simulink model "modules_intentions"  (R2017a)
settings: Solver=ode4  StartTime=0.0  StopTime=time_stop  FixedStep=time_step  RelTol=1e-3
undefined symbols (not defined in the file or in its folder): beta, Delta_guidance, Delta_matrix, eta_initial, initial_desired_psi_vector, initial_desired_u_vector, initial_next_waypoint_indexes, initial_obstacle_ship_states, initial_obstacle_ship_states_dot, initial_reference_psi_vector, initial_reference_u_vector, initial_SBMPC_desired_psi_vector, initial_SBMPC_desired_u_vector, initial_SBMPC_next_waypoint_indexes, initial_SBMPC_obstacle_ship_states, initial_SBMPC_obstacle_ship_states_dot, initial_SBMPC_reference_psi_vector, initial_SBMPC_reference_u_vector, initial_SBMPC_x_d_psi_matrix, initial_SBMPC_x_d_u_matrix, initial_state, initial_x_d_psi_matrix, initial_x_d_u_matrix, K_sway, K_yaw, Kp_feedback_linearization, kp_heading, Nmax, nu_initial, num_obs_ship_waypoints, num_prediction_time_steps, number_of_control_behaviors, number_of_obstacle_ships, number_of_SBMPC_obstacle_ships, obs_speed_between_waypoints, obstacle_waypoint_matrix, Omega_matrix, own_ship_reference_psi_init, own_ship_reference_speed, psi, Psi_init, radius_of_acceptance, SBMPC_obs_speed_between_waypoints, SBMPC_obstacle_waypoint_matrix, seconds_between_prediction, state_vector_init, T, T_k_surge, T_k_sway, T_k_yaw, T_s, T_waypoints, time_step, tsamp, U, U_init, V_init, waypoints_obstacle_ships, waypoints_own_ship, Xmax ... (+1)
(part 2 of 6)

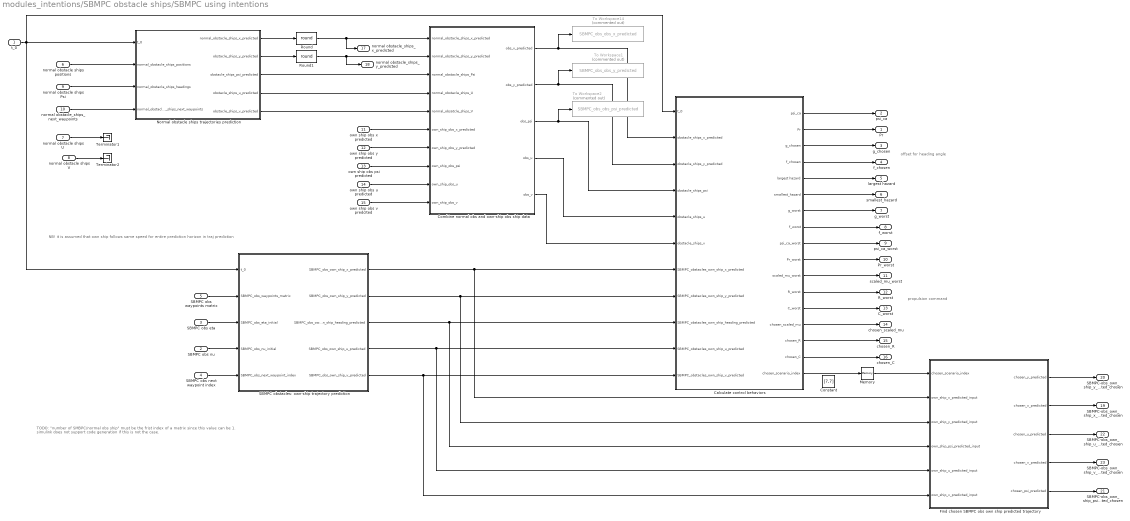
== system modules_intentions/SBMPC obstacle ships/SBMPC using intentions  ==
  note: TODO: "number of SMBPC/normal obs ship" must be the frist index of a matrix since this value can be 1. simulink
      | does not support code generation if this is not the case.
  note: propulsion command
  note: offset for heading angle
  note: NB! it is assumed that own ship follows same speed for entire prediction horizon in traj prediction
  t_0 : Inport
  SBMPC obs nu : Inport  Port=2
  SBMPC obs eta : Inport  Port=3
  SBMPC obs next waypoint index : Inport  Port=4
  "SBMPC obs waypoints matrix " : Inport  Port=5
  normal obstacle ships positions : Inport  Port=6
  normal obstacle ships U : Inport  Port=7
  normal obstacle ships V : Inport  Port=8
  normal obstacle ships Psi : Inport  Port=9
  normal obstacle_ships_next_waypoints : Inport  Port=10
  own ship obs x predicted : Inport  Port=11  SampleTime=time_step
  own ship obs y predicted : Inport  Port=12  SampleTime=time_step
  own ship obs psi predicted : Inport  Port=13
  own ship obs u predicted : Inport  Port=14
  own ship obs v predcited : Inport  Port=15
  Calculate control behaviors : Subsystem
  "Combine normal obs and own-ship obs ship data " : MATLAB Function  TreatAsAtomicUnit=on
  Constant : Constant  Value=[7,7]  VectorParams1D=off
  Find chosen SBMPC obs own ship predicted trajectory : MATLAB Function  TreatAsAtomicUnit=on
  Memory : Memory  X0=7
  Normal obstacle ships trajectories prediction : Subsystem
  Round : Rounding  Operator=round
  Round1 : Rounding  Operator=round
  SBMPC obstacles: own-ship trajectory prediction : Subsystem
  Terminator1 : Terminator
  Terminator2 : Terminator
  To Workspace1 : ToWorkspace  Commented=on  VariableName=SBMPC_obs_obs_y_predicted  SaveFormat=Structure With Time  SampleTime=tsamp
      settings: Save2DSignal=2-D array (concatenate along first dimension)
  To Workspace14 : ToWorkspace  Commented=on  VariableName=SBMPC_obs_obs_x_predicted  SaveFormat=Structure With Time  SampleTime=tsamp
      settings: Save2DSignal=2-D array (concatenate along first dimension)
  To Workspace2 : ToWorkspace  Commented=on  VariableName=SBMPC_obs_obs_psi_predicted  SaveFormat=Structure With Time  SampleTime=tsamp
      settings: Save2DSignal=2-D array (concatenate along first dimension)
  Pr : Outport
  psi_ca : Outport  Port=2
  "g_chosen " : Outport  Port=3  SampleTime=time_step
  f_chosen : Outport  Port=4  SampleTime=time_step
  largest hazard : Outport  Port=5  SampleTime=time_step
  smallest_hazard : Outport  Port=6  SampleTime=time_step
  "g_worst " : Outport  Port=7  SampleTime=time_step
  f_worst : Outport  Port=8  SampleTime=time_step
  psi_ca_worst : Outport  Port=9  SampleTime=time_step
  Pr_worst : Outport  Port=10  SampleTime=time_step
  scaled_mu_worst : Outport  Port=11  SampleTime=time_step
  R_worst : Outport  Port=12  SampleTime=time_step
  C_worst : Outport  Port=13  SampleTime=time_step
  chosen_scaled_mu : Outport  Port=14  SampleTime=time_step
  chosen_R : Outport  Port=15  SampleTime=time_step
  chosen_C : Outport  Port=16  SampleTime=time_step
  normal obstacle_ships_x_predicted : Outport  Port=17  SampleTime=time_step
  "normal obstacle_ships_y_predicted " : Outport  Port=18  SampleTime=time_step
  SBMPC-obs_own_ship_x_predicted_chosen : Outport  Port=19  SampleTime=time_step
  SBMPC-obs_own_ship_y_predicted_chosen : Outport  Port=20  SampleTime=time_step
  SBMPC-obs_own_ship_psi_predicted_chosen : Outport  Port=21  SampleTime=time_step
  SBMPC-obs_own_ship_u_predicted_chosen : Outport  Port=22  SampleTime=time_step
  SBMPC-obs_own_ship_v_predicted_chosen : Outport  Port=23  SampleTime=time_step
  wires:
  "SBMPC obs waypoints matrix "/1 -> SBMPC obstacles: own-ship trajectory prediction/2(SBMPC_obs_waypoints_matrix)
  SBMPC obs eta/1 -> SBMPC obstacles: own-ship trajectory prediction/3("SBMPC_obs_eta_initial ")
  SBMPC obs nu/1 -> SBMPC obstacles: own-ship trajectory prediction/4(SBMPC_obs_nu_initial)
  SBMPC obs next waypoint index/1 -> SBMPC obstacles: own-ship trajectory prediction/5(SBMPC_obs_next_waypoint_index)
  t_0/1 -> Calculate control behaviors/1(t_0), Normal obstacle ships trajectories prediction/1(t_0), SBMPC obstacles: own-ship trajectory prediction/1(t_0)
  normal obstacle ships positions/1 -> Normal obstacle ships trajectories prediction/2(normal_obstacle_ships_positions)
  normal obstacle ships Psi/1 -> Normal obstacle ships trajectories prediction/3(normal_obstacle_ships_headings)
  SBMPC obstacles: own-ship trajectory prediction/5("SBMPC_obs_own_ship_v_predicted ") -> Find chosen SBMPC obs own ship predicted trajectory/6(own_ship_v_predicted_input), Calculate control behaviors/11("SBMPC_obstacles_own_ship_v_predicted ")
  SBMPC obstacles: own-ship trajectory prediction/3(SBMPC_obs_own_ship_heading_predicted) -> Calculate control behaviors/9("SBMPC_obstacles_own_ship_heading_predicted "), Find chosen SBMPC obs own ship predicted trajectory/4(own_ship_psi_predicted_input)
  Calculate control behaviors/2(Pr) -> Pr/1
  Calculate control behaviors/1(psi_ca) -> psi_ca/1
  normal obstacle_ships_next_waypoints/1 -> Normal obstacle ships trajectories prediction/4(normal_obstacle_ships_next_waypoints)
  Calculate control behaviors/16(chosen_C) -> chosen_C/1
  Calculate control behaviors/15(chosen_R) -> chosen_R/1
  Calculate control behaviors/14(chosen_scaled_mu) -> chosen_scaled_mu/1
  Calculate control behaviors/13(C_worst) -> C_worst/1
  Calculate control behaviors/12(R_worst) -> R_worst/1
  Calculate control behaviors/11(scaled_mu_worst) -> scaled_mu_worst/1
  Calculate control behaviors/10(Pr_worst) -> Pr_worst/1
  Calculate control behaviors/9(psi_ca_worst) -> psi_ca_worst/1
  Calculate control behaviors/8(f_worst) -> f_worst/1
  Calculate control behaviors/7("g_worst ") -> "g_worst "/1
  Calculate control behaviors/6(smallest_hazard) -> smallest_hazard/1
  Calculate control behaviors/5(largest hazard) -> largest hazard/1
  Calculate control behaviors/4(f_chosen) -> f_chosen/1
  Calculate control behaviors/3("g_chosen ") -> "g_chosen "/1
  "Combine normal obs and own-ship obs ship data "/5(obs_v) -> Calculate control behaviors/6(obstacle_ships_v)
  "Combine normal obs and own-ship obs ship data "/4(obs_u) -> Calculate control behaviors/5(obstacle_ships_u)
  "Combine normal obs and own-ship obs ship data "/3(obs_psi) -> To Workspace2/1, Calculate control behaviors/4(obstacle_ships_psi)
  "Combine normal obs and own-ship obs ship data "/2(obs_y_predicted) -> To Workspace1/1, Calculate control behaviors/3("obstacle_ships_y_predicted ")
  "Combine normal obs and own-ship obs ship data "/1(obs_x_predicted) -> To Workspace14/1, Calculate control behaviors/2(obstacle_ships_x_predicted)
  own ship obs x predicted/1 -> "Combine normal obs and own-ship obs ship data "/6(own_ship_obs_x_predicted)
  own ship obs y predicted/1 -> "Combine normal obs and own-ship obs ship data "/7(own_ship_obs_y_predicted)
  own ship obs psi predicted/1 -> "Combine normal obs and own-ship obs ship data "/8(own_ship_obs_psi)
  own ship obs u predicted/1 -> "Combine normal obs and own-ship obs ship data "/9(own_ship_obs_u)
  own ship obs v predcited/1 -> "Combine normal obs and own-ship obs ship data "/10(own_ship_obs_v)
  SBMPC obstacles: own-ship trajectory prediction/1(SBMPC_obs_own_ship_x_predicted) -> Find chosen SBMPC obs own ship predicted trajectory/2(own_ship_x_predicted_input), Calculate control behaviors/7(SBMPC_obstacles_own_ship_x_predicted)
  SBMPC obstacles: own-ship trajectory prediction/2(SBMPC_obs_own_ship_y_predicted) -> Find chosen SBMPC obs own ship predicted trajectory/3(own_ship_y_predicted_input), Calculate control behaviors/8(SBMPC_obstacles_own_ship_y_predicted)
  SBMPC obstacles: own-ship trajectory prediction/4(SBMPC_obs_own_ship_u_predicted) -> Find chosen SBMPC obs own ship predicted trajectory/5(own_ship_u_predicted_input), Calculate control behaviors/10(SBMPC_obstacles_own_ship_u_predicted)
  Memory/1 -> Find chosen SBMPC obs own ship predicted trajectory/1(chosen_scenario_index)
  Find chosen SBMPC obs own ship predicted trajectory/1(chosen_y_predicted) -> SBMPC-obs_own_ship_y_predicted_chosen/1
  Find chosen SBMPC obs own ship predicted trajectory/2(chosen_x_predicted) -> SBMPC-obs_own_ship_x_predicted_chosen/1
  Find chosen SBMPC obs own ship predicted trajectory/3(chosen_u_predicted) -> SBMPC-obs_own_ship_u_predicted_chosen/1
  Find chosen SBMPC obs own ship predicted trajectory/4(chosen_v_predicted) -> SBMPC-obs_own_ship_v_predicted_chosen/1
  Find chosen SBMPC obs own ship predicted trajectory/5(chosen_psi_predicted) -> SBMPC-obs_own_ship_psi_predicted_chosen/1
  Normal obstacle ships trajectories prediction/2(obstacle_ships_y_predicted) -> Round1/1
  Normal obstacle ships trajectories prediction/3(obstacle_ships_psi_predicted) -> "Combine normal obs and own-ship obs ship data "/3(normal_obstacle_ships_Psi)
  Normal obstacle ships trajectories prediction/4(obstacle_ships_u_predicted) -> "Combine normal obs and own-ship obs ship data "/4(normal_obstacle_ships_U)
  Normal obstacle ships trajectories prediction/5(obstacle_ships_v_predicted) -> "Combine normal obs and own-ship obs ship data "/5(normal_obsatcle_ships_V)
  Normal obstacle ships trajectories prediction/1(normal_obstacle_ships_x_predicted) -> Round/1
  normal obstacle ships U/1 -> Terminator1/1
  normal obstacle ships V/1 -> Terminator2/1
  Calculate control behaviors/17(chosen_scenario_index) -> Memory/1
  Round/1 -> normal obstacle_ships_x_predicted/1, "Combine normal obs and own-ship obs ship data "/1(normal_obstacle_ships_x_predicted)
  Round1/1 -> "normal obstacle_ships_y_predicted "/1, "Combine normal obs and own-ship obs ship data "/2(normal_obstacle_ships_y_predicted)

== system modules_intentions/SBMPC obstacle ships/guidance  ==
  state matrix : Inport
  "waypoints matrix " : Inport  Port=2
  SBMPC obstacle waypoint guidance : MATLAB Function  TreatAsAtomicUnit=on
  SBMPC reference u vector : MATLAB Function  TreatAsAtomicUnit=on
  Scope : Scope
  Scope1 : Scope
  Scope2 : Scope
  "reference psi " : Outport
  reference u vector : Outport  Port=2
  "next_waypoints_indexes " : Outport  Port=3
  wires:
  "waypoints matrix "/1 -> SBMPC obstacle waypoint guidance/1(SBMPC_obstacle_waypoints)
  state matrix/1 -> SBMPC obstacle waypoint guidance/2(state_matrix)
  SBMPC obstacle waypoint guidance/1(reference_psi_vector) -> "reference psi "/1, Scope/1
  SBMPC reference u vector/1(u_vector) -> Scope2/1, reference u vector/1
  SBMPC obstacle waypoint guidance/2(next_waypoints_indexes) -> SBMPC reference u vector/1(next_waypoints_indexes), Scope1/1, "next_waypoints_indexes "/1

== system modules_intentions/SBMPC obstacle ships/reference model for psi ==
  note: row vector
  note: row vector
  reference psi vector : Inport
  "SBMPC psi reference model " : MATLAB Function  TreatAsAtomicUnit=on
  Scope3 : Scope  NumInputPorts=2
  To Workspace : ToWorkspace  VariableName=SBMPC_obstacle_ships_reference_psi_vector  SampleTime=tsamp
      settings: Save2DSignal=2-D array (concatenate along first dimension)
  To Workspace1 : ToWorkspace  VariableName=SBMPC_obstacle_ships_desired_psi_vector  SampleTime=tsamp
      settings: Save2DSignal=2-D array (concatenate along first dimension)
  "desired psi vector " : Outport
  wires:
  "SBMPC psi reference model "/1(desired_psi_vector) -> Scope3/1, To Workspace1/1, "desired psi vector "/1
  reference psi vector/1 -> Scope3/2, To Workspace/1, "SBMPC psi reference model "/1(reference_psi_vector)

== system modules_intentions/SBMPC obstacle ships/reference model for u ==
  note: row vector
  note: row vector
  "reference u vector " : Inport
  SBMPC obstacle ships reference model u : MATLAB Function  TreatAsAtomicUnit=on
  To Workspace : ToWorkspace  VariableName=SBMPC_obstacle_ships_reference_u_vector  SampleTime=tsamp
      settings: Save2DSignal=2-D array (concatenate along first dimension)
  To Workspace1 : ToWorkspace  VariableName=SBMPC_obstacle_ships_desired_u_vector  SampleTime=tsamp
      settings: Save2DSignal=2-D array (concatenate along first dimension)
  desired_u_vector : Outport
  wires:
  "reference u vector "/1 -> To Workspace/1, SBMPC obstacle ships reference model u/1(reference_u_vetor)
  SBMPC obstacle ships reference model u/1(desired_u_vector) -> To Workspace1/1, desired_u_vector/1

== system modules_intentions/normal obstacle ships/guidance  ==
  state matrix : Inport
  "waypoints matrix " : Inport  Port=2
  MATLAB Function1 : MATLAB Function  TreatAsAtomicUnit=on
  Scope : Scope
  Scope1 : Scope
  Scope2 : Scope
  obstacle waypoint guidance : MATLAB Function  TreatAsAtomicUnit=on
  "reference psi " : Outport
  reference u vector : Outport  Port=2
  "next_waypoints_indexes " : Outport  Port=3
  wires:
  "waypoints matrix "/1 -> obstacle waypoint guidance/1(obstacle_waypoints)
  state matrix/1 -> obstacle waypoint guidance/2(state_matrix)
  obstacle waypoint guidance/1(reference_psi_vector) -> "reference psi "/1, Scope/1
  MATLAB Function1/1(u_vector) -> Scope2/1, reference u vector/1
  obstacle waypoint guidance/2(next_waypoints_indexes) -> MATLAB Function1/1(next_waypoints_indexes), Scope1/1, "next_waypoints_indexes "/1

== system modules_intentions/normal obstacle ships/reference model for psi ==
  note: row vector
  note: row vector
  reference psi vector : Inport
  Scope3 : Scope  NumInputPorts=2
  To Workspace : ToWorkspace  VariableName=obstacle_ships_reference_psi_vector  SampleTime=tsamp
      settings: Save2DSignal=2-D array (concatenate along first dimension)
  To Workspace1 : ToWorkspace  VariableName=obstacle_ships_desired_psi_vector  SampleTime=tsamp
      settings: Save2DSignal=2-D array (concatenate along first dimension)
  "psi reference model " : MATLAB Function  TreatAsAtomicUnit=on
  "desired psi vector " : Outport
  wires:
  "psi reference model "/1(desired_psi_vector) -> Scope3/1, To Workspace1/1, "desired psi vector "/1
  reference psi vector/1 -> Scope3/2, To Workspace/1, "psi reference model "/1(reference_psi_vector)

== system modules_intentions/normal obstacle ships/reference model for u ==
  note: row vector
  note: row vector
  "reference u vector " : Inport
  MATLAB Function1 : MATLAB Function  TreatAsAtomicUnit=on
  To Workspace : ToWorkspace  VariableName=obstacle_ships_reference_u_vector  SampleTime=tsamp
      settings: Save2DSignal=2-D array (concatenate along first dimension)
  To Workspace1 : ToWorkspace  VariableName=obstacle_ships_desired_u_vector  SampleTime=tsamp
      settings: Save2DSignal=2-D array (concatenate along first dimension)
  desired_u_vector : Outport
  wires:
  "reference u vector "/1 -> To Workspace/1, MATLAB Function1/1(reference_u_vetor)
  MATLAB Function1/1(desired_u_vector) -> To Workspace1/1, desired_u_vector/1

== system modules_intentions/Own-ship/Own-ship PSV/PSV ==
  desired_nu : Inport
  desired_psi : Inport  Port=2
  Pr : Inport  Port=3
  psi_ca : Inport  Port=4
  Demux : Demux  Outputs=6
  Mux : Mux  Inputs=3
  PSV model : MATLAB Function  TreatAsAtomicUnit=on
  Terminator : Terminator
  To Workspace : ToWorkspace  VariableName=tau  SampleTime=tsamp
      settings: Save2DSignal=2-D array (concatenate along first dimension)
  state : Outport
  x : Outport  Port=2
  y : Outport  Port=3
  psi : Outport  Port=4
  u : Outport  Port=5
  v : Outport  Port=6
  r : Outport  Port=7
  wires:
  Demux/4 -> u/1, Mux/1
  Mux/1 -> Terminator/1  "nu"
  PSV model/1(state) -> Demux/1, state/1
  Demux/5 -> v/1, Mux/2
  Demux/2 -> y/1
  Demux/6 -> r/1, Mux/3
  Demux/1 -> x/1
  Demux/3 -> psi/1
  desired_psi/1 -> PSV model/4(desired_psi)
  desired_nu/1 -> PSV model/3(desired_nu)
  PSV model/2(tau) -> To Workspace/1
  psi_ca/1 -> PSV model/2(psi_ca)
  Pr/1 -> PSV model/1(Pr)

== system modules_intentions/Own-ship/Own-ship PSV/derivative ==
  desired_nu : Inport
  Memory2 : Memory
  vector derivative : MATLAB Function  TreatAsAtomicUnit=on
  desired_nu_dot : Outport
  wires:
  Memory2/1 -> vector derivative/2(x_previous)
  desired_nu/1 -> Memory2/1, vector derivative/1(x)
  vector derivative/1(derivative) -> desired_nu_dot/1

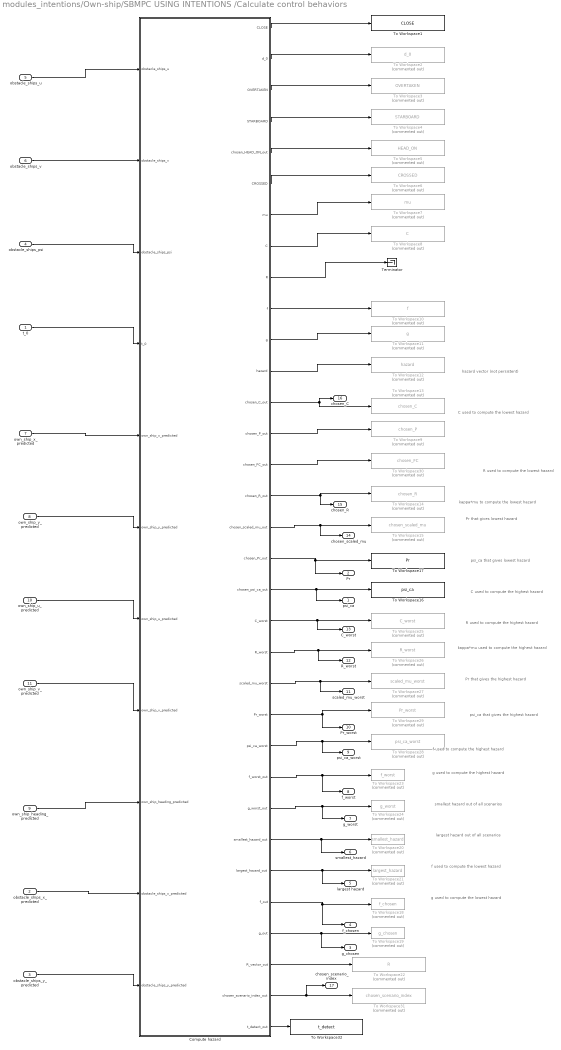
== system modules_intentions/Own-ship/SBMPC USING INTENTIONS /Calculate control behaviors ==
  note: hazard vector (not persistent)
  note: C used to compute the lowest hazard
  note: R used to compute the lowest hazard
  note: kappa*mu to compute the lowest hazard
  note: Pr that gives lowest hazard
  note: psi_ca that gives lowest hazard
  note: C used to compute the highest hazard
  note: R used to compute the highest hazard
  note: kappa*mu used to compute the highest hazard
  note: Pr that gives the highest hazard
  note: psi_ca that gives the highest hazard
  note: f used to compute the highest hazard
  note: g used to compute the highest hazard
  note: smallest hazard out of all scenarios
  note: largest hazard out of all scenarios
  note: f used to compute the lowest hazard
  note: g used to compute the lowest hazard
  t_0 : Inport
  obstacle_ships_x_predicted : Inport  Port=2  SampleTime=time_step
      settings: VarSizeSig=Yes
  "obstacle_ships_y_predicted " : Inport  Port=3  SampleTime=time_step
      settings: VarSizeSig=Yes
  obstacle_ships_psi : Inport  Port=4
  obstacle_ships_u : Inport  Port=5
  obstacle_ships_v : Inport  Port=6
  own_ship_x_predicted : Inport  Port=7  SampleTime=time_step
      settings: VarSizeSig=Yes
  own_ship_y_predicted : Inport  Port=8  SampleTime=time_step
      settings: VarSizeSig=Yes
  "own_ship_heading_predicted " : Inport  Port=9  SampleTime=time_step
      settings: VarSizeSig=Yes
  own_ship_u_predicted : Inport  Port=10  SampleTime=time_step
      settings: VarSizeSig=Yes
  "own_ship_v_predicted " : Inport  Port=11  SampleTime=time_step
      settings: VarSizeSig=Yes
  Compute hazard : MATLAB Function  TreatAsAtomicUnit=on
  Terminator : Terminator
  To Workspace1 : ToWorkspace  VariableName=CLOSE  SaveFormat=Structure With Time  SampleTime=tsamp
  To Workspace10 : ToWorkspace  Commented=on  VariableName=f  SaveFormat=Structure With Time  SampleTime=tsamp
      settings: Save2DSignal=2-D array (concatenate along first dimension)
  To Workspace11 : ToWorkspace  Commented=on  VariableName=g  SaveFormat=Structure With Time  SampleTime=tsamp
  To Workspace12 : ToWorkspace  Commented=on  VariableName=hazard  SaveFormat=Structure With Time  SampleTime=tsamp
      settings: Save2DSignal=2-D array (concatenate along first dimension)
  To Workspace13 : ToWorkspace  Commented=on  VariableName=chosen_C  SampleTime=tsamp
      settings: Save2DSignal=2-D array (concatenate along first dimension)
  To Workspace14 : ToWorkspace  Commented=on  VariableName=chosen_R  SampleTime=tsamp
      settings: Save2DSignal=2-D array (concatenate along first dimension)
  To Workspace15 : ToWorkspace  Commented=on  VariableName=chosen_scaled_mu  SampleTime=tsamp
      settings: Save2DSignal=2-D array (concatenate along first dimension)
  To Workspace16 : ToWorkspace  VariableName=psi_ca  SampleTime=tsamp
      settings: Save2DSignal=2-D array (concatenate along first dimension)
  To Workspace17 : ToWorkspace  VariableName=Pr  SampleTime=tsamp
      settings: Save2DSignal=2-D array (concatenate along first dimension)
  To Workspace18 : ToWorkspace  Commented=on  VariableName=f_chosen  SampleTime=tsamp
      settings: Save2DSignal=2-D array (concatenate along first dimension)
  To Workspace19 : ToWorkspace  Commented=on  VariableName=g_chosen  SampleTime=tsamp
      settings: Save2DSignal=2-D array (concatenate along first dimension)
  To Workspace2 : ToWorkspace  Commented=on  VariableName=d_0  SaveFormat=Structure With Time  SampleTime=tsamp
  To Workspace20 : ToWorkspace  Commented=on  VariableName=smallest_hazard  SampleTime=tsamp
      settings: Save2DSignal=2-D array (concatenate along first dimension)
  To Workspace21 : ToWorkspace  Commented=on  VariableName=largest_hazard  SampleTime=tsamp
      settings: Save2DSignal=2-D array (concatenate along first dimension)
  To Workspace22 : ToWorkspace  Commented=on  VariableName=R  SaveFormat=Structure With Time  SampleTime=tsamp
  To Workspace23 : ToWorkspace  Commented=on  VariableName=f_worst  SampleTime=tsamp
      settings: Save2DSignal=2-D array (concatenate along first dimension)
  To Workspace24 : ToWorkspace  Commented=on  VariableName=g_worst  SampleTime=tsamp
      settings: Save2DSignal=2-D array (concatenate along first dimension)
  To Workspace25 : ToWorkspace  Commented=on  VariableName=C_worst  SampleTime=tsamp
      settings: Save2DSignal=2-D array (concatenate along first dimension)
  To Workspace26 : ToWorkspace  Commented=on  VariableName=R_worst  SampleTime=tsamp
      settings: Save2DSignal=2-D array (concatenate along first dimension)
  To Workspace27 : ToWorkspace  Commented=on  VariableName=scaled_mu_worst  SampleTime=tsamp
      settings: Save2DSignal=2-D array (concatenate along first dimension)
  To Workspace28 : ToWorkspace  Commented=on  VariableName=psi_ca_worst  SampleTime=tsamp
      settings: Save2DSignal=2-D array (concatenate along first dimension)
  To Workspace29 : ToWorkspace  Commented=on  VariableName=Pr_worst  SampleTime=tsamp
      settings: Save2DSignal=2-D array (concatenate along first dimension)
  To Workspace3 : ToWorkspace  Commented=on  VariableName=OVERTAKEN  SampleTime=tsamp
  To Workspace30 : ToWorkspace  Commented=on  VariableName=chosen_FC  SampleTime=tsamp
      settings: Save2DSignal=2-D array (concatenate along first dimension)
  To Workspace31 : ToWorkspace  Commented=on  VariableName=chosen_scenario_index  SampleTime=tsamp
      settings: Save2DSignal=2-D array (concatenate along first dimension)
  To Workspace32 : ToWorkspace  VariableName=t_detect  SaveFormat=Structure With Time  SampleTime=tsamp
      settings: Save2DSignal=2-D array (concatenate along first dimension)
  To Workspace4 : ToWorkspace  Commented=on  VariableName=STARBOARD  SampleTime=tsamp
  To Workspace5 : ToWorkspace  Commented=on  VariableName=HEAD_ON  SampleTime=tsamp
      settings: Save2DSignal=2-D array (concatenate along first dimension)
  To Workspace6 : ToWorkspace  Commented=on  VariableName=CROSSED  SampleTime=tsamp
  To Workspace7 : ToWorkspace  Commented=on  VariableName=mu  SaveFormat=Structure With Time  SampleTime=tsamp
  To Workspace8 : ToWorkspace  Commented=on  VariableName=C  SampleTime=tsamp
  To Workspace9 : ToWorkspace  Commented=on  VariableName=chosen_P  SampleTime=tsamp
      settings: Save2DSignal=2-D array (concatenate along first dimension)
  psi_ca : Outport  SampleTime=time_step
  Pr : Outport  Port=2  SampleTime=time_step
  "g_chosen " : Outport  Port=3  SampleTime=time_step
  f_chosen : Outport  Port=4  SampleTime=time_step
  largest hazard : Outport  Port=5  SampleTime=time_step
  smallest_hazard : Outport  Port=6  SampleTime=time_step
  "g_worst " : Outport  Port=7  SampleTime=time_step
  f_worst : Outport  Port=8  SampleTime=time_step
  psi_ca_worst : Outport  Port=9  SampleTime=time_step
  Pr_worst : Outport  Port=10  SampleTime=time_step
  scaled_mu_worst : Outport  Port=11  SampleTime=time_step
  R_worst : Outport  Port=12  SampleTime=time_step
  C_worst : Outport  Port=13  SampleTime=time_step
  chosen_scaled_mu : Outport  Port=14  SampleTime=time_step
  chosen_R : Outport  Port=15  SampleTime=time_step
  chosen_C : Outport  Port=16  SampleTime=time_step
  "chosen_scenario_index " : Outport  Port=17  SampleTime=time_step
  wires:
  own_ship_x_predicted/1 -> Compute hazard/5(own_ship_x_predicted)
  own_ship_y_predicted/1 -> Compute hazard/6(own_ship_y_predicted)
  obstacle_ships_x_predicted/1 -> Compute hazard/10(obstacle_ships_x_predicted)
  "obstacle_ships_y_predicted "/1 -> Compute hazard/11(obstacle_ships_y_predicted)
  t_0/1 -> Compute hazard/4(t_0)
  Compute hazard/1(CLOSE) -> To Workspace1/1
  Compute hazard/2(d_0) -> To Workspace2/1
  obstacle_ships_v/1 -> Compute hazard/2(obstacle_ships_v)
  obstacle_ships_u/1 -> Compute hazard/1(obstacle_ships_u)
  own_ship_u_predicted/1 -> Compute hazard/7(own_ship_u_predicted)
  "own_ship_v_predicted "/1 -> Compute hazard/8(own_ship_v_predicted)
  "own_ship_heading_predicted "/1 -> Compute hazard/9(own_ship_heading_predicted)
  obstacle_ships_psi/1 -> Compute hazard/3(obstacle_ships_psi)
  Compute hazard/3(OVERTAKEN) -> To Workspace3/1
  Compute hazard/4(STARBOARD) -> To Workspace4/1
  Compute hazard/5(chosen_HEAD_ON_out) -> To Workspace5/1
  Compute hazard/6(CROSSED) -> To Workspace6/1
  Compute hazard/7(mu) -> To Workspace7/1
  Compute hazard/12(hazard) -> To Workspace12/1
  Compute hazard/8(C) -> To Workspace8/1
  Compute hazard/10(f) -> To Workspace10/1
  Compute hazard/11(g) -> To Workspace11/1
  Compute hazard/13(chosen_C_out) -> To Workspace13/1, chosen_C/1
  Compute hazard/16(chosen_R_out) -> chosen_R/1, To Workspace14/1
  Compute hazard/17(chosen_scaled_mu_out) -> chosen_scaled_mu/1, To Workspace15/1
  Compute hazard/19(chosen_psi_ca_out) -> psi_ca/1, To Workspace16/1
  Compute hazard/20(C_worst) -> C_worst/1, To Workspace25/1
  Compute hazard/21(R_worst) -> R_worst/1, To Workspace26/1
  Compute hazard/22(scaled_mu_worst) -> scaled_mu_worst/1, To Workspace27/1
  Compute hazard/23(Pr_worst) -> Pr_worst/1, To Workspace29/1
  Compute hazard/24(psi_ca_worst) -> psi_ca_worst/1, To Workspace28/1
  Compute hazard/26(g_worst_out) -> "g_worst "/1, To Workspace24/1
  Compute hazard/25(f_worst_out) -> f_worst/1, To Workspace23/1
  Compute hazard/18(chosen_Pr_out) -> Pr/1, To Workspace17/1
  Compute hazard/29(f_out) -> f_chosen/1, To Workspace18/1
  Compute hazard/30(g_out) -> "g_chosen "/1, To Workspace19/1
  Compute hazard/27(smallest_hazard_out) -> smallest_hazard/1, To Workspace20/1
  Compute hazard/28(largest_hazard_out) -> largest hazard/1, To Workspace21/1
  Compute hazard/31(R_vector_out) -> To Workspace22/1
  Compute hazard/9(R) -> Terminator/1
  Compute hazard/14(chosen_P_out) -> To Workspace9/1
  Compute hazard/15(chosen_FC_out) -> To Workspace30/1
  Compute hazard/32(chosen_scenario_index_out) -> "chosen_scenario_index "/1, To Workspace31/1
  Compute hazard/33(t_detect_out) -> To Workspace32/1

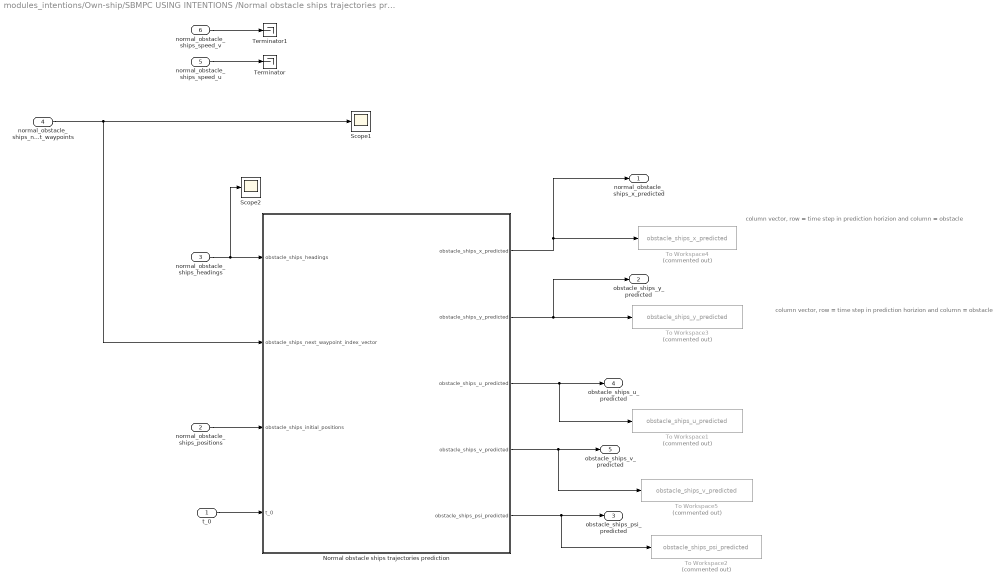
== system modules_intentions/Own-ship/SBMPC USING INTENTIONS /Normal obstacle ships trajectories prediction ==
  note: column vector, row = time step in prediction horizion and column = obstacle
  note: column vector, row = time step in prediction horizion and column = obstacle
  t_0 : Inport
  normal_obstacle_ships_positions : Inport  Port=2
  normal_obstacle_ships_headings : Inport  Port=3
  normal_obstacle_ships_next_waypoints : Inport  Port=4
  normal_obstacle_ships_speed_u : Inport  Port=5
  normal_obstacle_ships_speed_v : Inport  Port=6
  Normal obstacle ships trajectories prediction : MATLAB Function  TreatAsAtomicUnit=on
  Scope1 : Scope
  Scope2 : Scope
  Terminator : Terminator
  Terminator1 : Terminator
  To Workspace1 : ToWorkspace  Commented=on  VariableName=obstacle_ships_u_predicted  SaveFormat=Structure With Time  SampleTime=tsamp
  To Workspace2 : ToWorkspace  Commented=on  VariableName=obstacle_ships_psi_predicted  SaveFormat=Structure With Time  SampleTime=tsamp
  To Workspace3 : ToWorkspace  Commented=on  VariableName=obstacle_ships_y_predicted  SaveFormat=Structure With Time  SampleTime=tsamp
  To Workspace4 : ToWorkspace  Commented=on  VariableName=obstacle_ships_x_predicted  SaveFormat=Structure With Time  SampleTime=tsamp
  To Workspace5 : ToWorkspace  Commented=on  VariableName=obstacle_ships_v_predicted  SaveFormat=Structure With Time  SampleTime=tsamp
  normal_obstacle_ships_x_predicted : Outport  SampleTime=time_step
  obstacle_ships_y_predicted : Outport  Port=2  SampleTime=time_step
  obstacle_ships_psi_predicted : Outport  Port=3  SampleTime=time_step
  obstacle_ships_u_predicted : Outport  Port=4  SampleTime=time_step
  obstacle_ships_v_predicted : Outport  Port=5  SampleTime=time_step
  wires:
  normal_obstacle_ships_positions/1 -> Normal obstacle ships trajectories prediction/3(obstacle_ships_initial_positions)
  normal_obstacle_ships_speed_v/1 -> Terminator1/1
  normal_obstacle_ships_speed_u/1 -> Terminator/1
  t_0/1 -> Normal obstacle ships trajectories prediction/4(t_0)
  Normal obstacle ships trajectories prediction/1(obstacle_ships_x_predicted) -> normal_obstacle_ships_x_predicted/1, To Workspace4/1
  Normal obstacle ships trajectories prediction/2(obstacle_ships_y_predicted) -> obstacle_ships_y_predicted/1, To Workspace3/1
  normal_obstacle_ships_headings/1 -> Scope2/1, Normal obstacle ships trajectories prediction/1(obstacle_ships_headings)
  normal_obstacle_ships_next_waypoints/1 -> Normal obstacle ships trajectories prediction/2(obstacle_ships_next_waypoint_index_vector), Scope1/1
  Normal obstacle ships trajectories prediction/3(obstacle_ships_u_predicted) -> To Workspace1/1, obstacle_ships_u_predicted/1
  Normal obstacle ships trajectories prediction/5(obstacle_ships_psi_predicted) -> To Workspace2/1, obstacle_ships_psi_predicted/1
  Normal obstacle ships trajectories prediction/4(obstacle_ships_v_predicted) -> To Workspace5/1, obstacle_ships_v_predicted/1

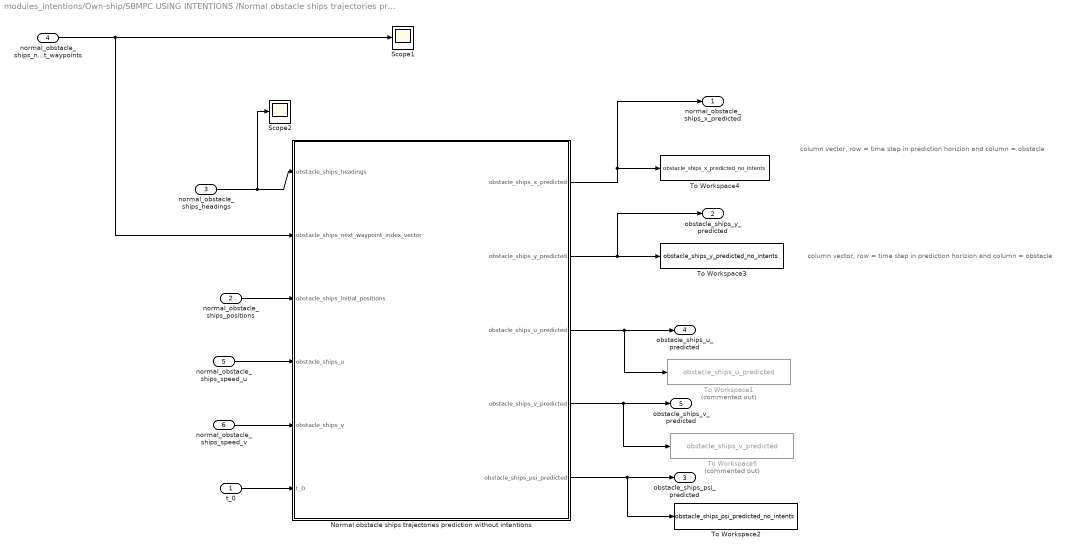
== system modules_intentions/Own-ship/SBMPC USING INTENTIONS /Normal obstacle ships trajectories prediction without intentions  ==
  note: column vector, row = time step in prediction horizion and column = obstacle
  note: column vector, row = time step in prediction horizion and column = obstacle
  t_0 : Inport
  normal_obstacle_ships_positions : Inport  Port=2
  normal_obstacle_ships_headings : Inport  Port=3
  normal_obstacle_ships_next_waypoints : Inport  Port=4
  normal_obstacle_ships_speed_u : Inport  Port=5
  normal_obstacle_ships_speed_v : Inport  Port=6
  Normal obstacle ships trajectories prediction without intentions : MATLAB Function  TreatAsAtomicUnit=on
  Scope1 : Scope
  Scope2 : Scope
  To Workspace1 : ToWorkspace  Commented=on  VariableName=obstacle_ships_u_predicted  SaveFormat=Structure With Time  SampleTime=tsamp
  To Workspace2 : ToWorkspace  VariableName=obstacle_ships_psi_predicted_no_intents  SaveFormat=Structure With Time  SampleTime=tsamp
  To Workspace3 : ToWorkspace  VariableName=obstacle_ships_y_predicted_no_intents  SaveFormat=Structure With Time  SampleTime=tsamp
  To Workspace4 : ToWorkspace  VariableName=obstacle_ships_x_predicted_no_intents  SaveFormat=Structure With Time  SampleTime=tsamp
  To Workspace5 : ToWorkspace  Commented=on  VariableName=obstacle_ships_v_predicted  SaveFormat=Structure With Time  SampleTime=tsamp
  normal_obstacle_ships_x_predicted : Outport  SampleTime=time_step
  obstacle_ships_y_predicted : Outport  Port=2  SampleTime=time_step
  obstacle_ships_psi_predicted : Outport  Port=3  SampleTime=time_step
  obstacle_ships_u_predicted : Outport  Port=4  SampleTime=time_step
  obstacle_ships_v_predicted : Outport  Port=5  SampleTime=time_step
  wires:
  normal_obstacle_ships_positions/1 -> Normal obstacle ships trajectories prediction without intentions/3(obstacle_ships_initial_positions)
  normal_obstacle_ships_speed_v/1 -> Normal obstacle ships trajectories prediction without intentions/5(obstacle_ships_v)
  normal_obstacle_ships_speed_u/1 -> Normal obstacle ships trajectories prediction without intentions/4(obstacle_ships_u)
  t_0/1 -> Normal obstacle ships trajectories prediction without intentions/6(t_0)
  Normal obstacle ships trajectories prediction without intentions/1(obstacle_ships_x_predicted) -> normal_obstacle_ships_x_predicted/1, To Workspace4/1
  Normal obstacle ships trajectories prediction without intentions/2(obstacle_ships_y_predicted) -> obstacle_ships_y_predicted/1, To Workspace3/1
  normal_obstacle_ships_headings/1 -> Scope2/1, Normal obstacle ships trajectories prediction without intentions/1(obstacle_ships_headings)
  normal_obstacle_ships_next_waypoints/1 -> Normal obstacle ships trajectories prediction without intentions/2(obstacle_ships_next_waypoint_index_vector), Scope1/1
  Normal obstacle ships trajectories prediction without intentions/3(obstacle_ships_u_predicted) -> To Workspace1/1, obstacle_ships_u_predicted/1
  Normal obstacle ships trajectories prediction without intentions/5(obstacle_ships_psi_predicted) -> To Workspace2/1, obstacle_ships_psi_predicted/1
  Normal obstacle ships trajectories prediction without intentions/4(obstacle_ships_v_predicted) -> To Workspace5/1, obstacle_ships_v_predicted/1

== system modules_intentions/Own-ship/SBMPC USING INTENTIONS /Own-ship trajectory prediction ==
  note: each row = time step in prediction horizion
      | each column = a different control scenario
  note: each row = time step in prediction horizion
      | each column = a different control scenario
  note: each row = time step in prediction horizion
      | each column = a different control scenario
  note: each row = time step in prediction horizion
      | each column = a different control scenario
  note: each row = time step in prediction horizion
      | each column = a different control scenario
  t_0 : Inport
  waypoints_matrix : Inport  Port=2
  "eta_initial " : Inport  Port=3
  nu_initial : Inport  Port=4
  next_waypoint_index : Inport  Port=5
  Own ship trajectory prediction : MATLAB Function  TreatAsAtomicUnit=on
  To Workspace1 : ToWorkspace  Commented=on  VariableName=own_ship_x_predicted  SaveFormat=Structure With Time  SampleTime=tsamp
  To Workspace3 : ToWorkspace  Commented=on  VariableName=own_ship_y_predicted  SaveFormat=Structure With Time  SampleTime=tsamp
  To Workspace4 : ToWorkspace  Commented=on  VariableName=own_ship_heading_predicted  SaveFormat=Structure With Time  SampleTime=tsamp
  To Workspace5 : ToWorkspace  Commented=on  VariableName=own_ship_u_predicted  SaveFormat=Structure With Time  SampleTime=tsamp
  To Workspace6 : ToWorkspace  Commented=on  VariableName=own_ship_v_predicted  SaveFormat=Structure With Time  SampleTime=tsamp
  own_ship_x_predicted : Outport  SampleTime=time_step
  own_ship_y_predicted : Outport  Port=2  SampleTime=time_step
  own_ship_heading_predicted : Outport  Port=3  SampleTime=time_step
  own_ship_u_predicted : Outport  Port=4  SampleTime=time_step
  "own_ship_v_predicted " : Outport  Port=5  SampleTime=time_step
  wires:
  waypoints_matrix/1 -> Own ship trajectory prediction/4(waypoints_matrix)
  nu_initial/1 -> Own ship trajectory prediction/3(nu_initial)
  "eta_initial "/1 -> Own ship trajectory prediction/2(eta_initial)
  next_waypoint_index/1 -> Own ship trajectory prediction/5(next_waypoint_index)
  t_0/1 -> Own ship trajectory prediction/1(t_0)
  Own ship trajectory prediction/1(own_ship_x_predicted) -> own_ship_x_predicted/1, To Workspace1/1
  Own ship trajectory prediction/2(own_ship_y_predicted) -> own_ship_y_predicted/1, To Workspace3/1
  Own ship trajectory prediction/3(own_ship_heading_predicted) -> To Workspace4/1, own_ship_heading_predicted/1
  Own ship trajectory prediction/4(own_ship_u_predicted) -> own_ship_u_predicted/1, To Workspace5/1
  Own ship trajectory prediction/5(own_ship_v_predicted) -> "own_ship_v_predicted "/1, To Workspace6/1

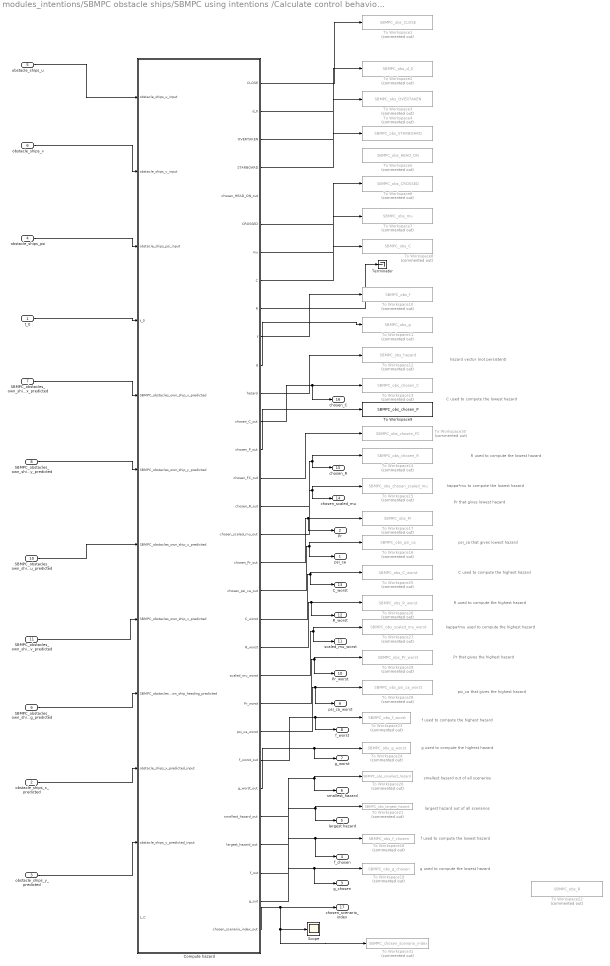
== system modules_intentions/SBMPC obstacle ships/SBMPC using intentions /Calculate control behaviors ==
  note: hazard vector (not persistent)
  note: C used to compute the lowest hazard
  note: R used to compute the lowest hazard
  note: kappa*mu to compute the lowest hazard
  note: Pr that gives lowest hazard
  note: psi_ca that gives lowest hazard
  note: C used to compute the highest hazard
  note: R used to compute the highest hazard
  note: kappa*mu used to compute the highest hazard
  note: Pr that gives the highest hazard
  note: psi_ca that gives the highest hazard
  note: f used to compute the highest hazard
  note: g used to compute the highest hazard
  note: smallest hazard out of all scenarios
  note: largest hazard out of all scenarios
  note: f used to compute the lowest hazard
  note: g used to compute the lowest hazard
  t_0 : Inport
  obstacle_ships_x_predicted : Inport  Port=2  SampleTime=time_step
      settings: VarSizeSig=Yes
  "obstacle_ships_y_predicted " : Inport  Port=3  SampleTime=time_step
      settings: VarSizeSig=Yes
  obstacle_ships_psi : Inport  Port=4
  obstacle_ships_u : Inport  Port=5
  obstacle_ships_v : Inport  Port=6
  SBMPC_obstacles_own_ship_x_predicted : Inport  Port=7  SampleTime=time_step
      settings: VarSizeSig=Yes
  SBMPC_obstacles_own_ship_y_predicted : Inport  Port=8  SampleTime=time_step
      settings: VarSizeSig=Yes
  "SBMPC_obstacles_own_ship_heading_predicted " : Inport  Port=9  SampleTime=time_step
      settings: VarSizeSig=Yes
  SBMPC_obstacles_own_ship_u_predicted : Inport  Port=10  SampleTime=time_step
      settings: VarSizeSig=Yes
  "SBMPC_obstacles_own_ship_v_predicted " : Inport  Port=11  SampleTime=time_step
      settings: VarSizeSig=Yes
  Compute hazard : MATLAB Function  TreatAsAtomicUnit=on
  Scope : Scope
  Terminator : Terminator
  To Workspace1 : ToWorkspace  Commented=on  VariableName=SBMPC_obs_CLOSE  SampleTime=tsamp
  To Workspace10 : ToWorkspace  Commented=on  VariableName=SBMPC_obs_f  SampleTime=tsamp
      settings: Save2DSignal=2-D array (concatenate along first dimension)
  To Workspace11 : ToWorkspace  Commented=on  VariableName=SBMPC_obs_g  SampleTime=tsamp
  To Workspace12 : ToWorkspace  Commented=on  VariableName=SBMPC_obs_hazard  SaveFormat=Structure With Time  SampleTime=tsamp
      settings: Save2DSignal=2-D array (concatenate along first dimension)
  To Workspace13 : ToWorkspace  Commented=on  VariableName=SBMPC_obs_chosen_C  SaveFormat=Structure With Time  SampleTime=tsamp
      settings: Save2DSignal=2-D array (concatenate along first dimension)
  To Workspace14 : ToWorkspace  Commented=on  VariableName=SBMPC_obs_chosen_R  SaveFormat=Structure With Time  SampleTime=tsamp
      settings: Save2DSignal=2-D array (concatenate along first dimension)
  To Workspace15 : ToWorkspace  Commented=on  VariableName=SBMPC_obs_chosen_scaled_mu  SaveFormat=Structure With Time  SampleTime=tsamp
      settings: Save2DSignal=2-D array (concatenate along first dimension)
  To Workspace16 : ToWorkspace  Commented=on  VariableName=SBMPC_obs_psi_ca  SaveFormat=Structure With Time  SampleTime=tsamp
      settings: Save2DSignal=2-D array (concatenate along first dimension)
  To Workspace17 : ToWorkspace  Commented=on  VariableName=SBMPC_obs_Pr  SaveFormat=Structure With Time  SampleTime=tsamp
      settings: Save2DSignal=2-D array (concatenate along first dimension)
  To Workspace18 : ToWorkspace  Commented=on  VariableName=SBMPC_obs_f_chosen  SaveFormat=Structure With Time  SampleTime=tsamp
      settings: Save2DSignal=2-D array (concatenate along first dimension)
  To Workspace19 : ToWorkspace  Commented=on  VariableName=SBMPC_obs_g_chosen  SaveFormat=Structure With Time  SampleTime=tsamp
      settings: Save2DSignal=2-D array (concatenate along first dimension)
  To Workspace2 : ToWorkspace  Commented=on  VariableName=SBMPC_obs_d_0  SampleTime=tsamp
  To Workspace20 : ToWorkspace  Commented=on  VariableName=SBMPC_obs_smallest_hazard  SaveFormat=Structure With Time  SampleTime=tsamp
      settings: Save2DSignal=2-D array (concatenate along first dimension)
  To Workspace21 : ToWorkspace  Commented=on  VariableName=SBMPC_obs_largest_hazard  SaveFormat=Structure With Time  SampleTime=tsamp
      settings: Save2DSignal=2-D array (concatenate along first dimension)
  To Workspace22 : ToWorkspace  Commented=on  VariableName=SBMPC_obs_R  SaveFormat=Structure With Time  SampleTime=tsamp
  To Workspace23 : ToWorkspace  Commented=on  VariableName=SBMPC_obs_f_worst  SaveFormat=Structure With Time  SampleTime=tsamp
      settings: Save2DSignal=2-D array (concatenate along first dimension)
  To Workspace24 : ToWorkspace  Commented=on  VariableName=SBMPC_obs_g_worst  SaveFormat=Structure With Time  SampleTime=tsamp
      settings: Save2DSignal=2-D array (concatenate along first dimension)
  To Workspace25 : ToWorkspace  Commented=on  VariableName=SBMPC_obs_C_worst  SaveFormat=Structure With Time  SampleTime=tsamp
      settings: Save2DSignal=2-D array (concatenate along first dimension)
  To Workspace26 : ToWorkspace  Commented=on  VariableName=SBMPC_obs_R_worst  SaveFormat=Structure With Time  SampleTime=tsamp
      settings: Save2DSignal=2-D array (concatenate along first dimension)
  To Workspace27 : ToWorkspace  Commented=on  VariableName=SBMPC_obs_scaled_mu_worst  SaveFormat=Structure With Time  SampleTime=tsamp
      settings: Save2DSignal=2-D array (concatenate along first dimension)
  To Workspace28 : ToWorkspace  Commented=on  VariableName=SBMPC_obs_psi_ca_worst  SaveFormat=Structure With Time  SampleTime=tsamp
      settings: Save2DSignal=2-D array (concatenate along first dimension)
  To Workspace29 : ToWorkspace  Commented=on  VariableName=SBMPC_obs_Pr_worst  SaveFormat=Structure With Time  SampleTime=tsamp
      settings: Save2DSignal=2-D array (concatenate along first dimension)
  To Workspace3 : ToWorkspace  Commented=on  VariableName=SBMPC_obs_OVERTAKEN  SampleTime=tsamp
  To Workspace30 : ToWorkspace  Commented=on  VariableName=SBMPC_obs_chosen_FC  SaveFormat=Structure With Time  SampleTime=tsamp
      settings: Save2DSignal=2-D array (concatenate along first dimension)
  To Workspace31 : ToWorkspace  Commented=on  VariableName=SBMPC_chosen_scenario_index  SaveFormat=Structure With Time  SampleTime=tsamp
      settings: Save2DSignal=2-D array (concatenate along first dimension)
  To Workspace4 : ToWorkspace  Commented=on  VariableName=SBMPC_obs_STARBOARD  SampleTime=tsamp
  To Workspace5 : ToWorkspace  Commented=on  VariableName=SBMPC_obs_HEAD_ON  SaveFormat=Structure With Time  SampleTime=tsamp
      settings: Save2DSignal=2-D array (concatenate along first dimension)
  To Workspace6 : ToWorkspace  Commented=on  VariableName=SBMPC_obs_CROSSED  SampleTime=tsamp
  To Workspace7 : ToWorkspace  Commented=on  VariableName=SBMPC_obs_mu  SampleTime=tsamp
  To Workspace8 : ToWorkspace  Commented=on  VariableName=SBMPC_obs_C  SampleTime=tsamp
  To Workspace9 : ToWorkspace  VariableName=SBMPC_obs_chosen_P  SaveFormat=Structure With Time  SampleTime=tsamp
      settings: Save2DSignal=2-D array (concatenate along first dimension)
  psi_ca : Outport  SampleTime=time_step
  Pr : Outport  Port=2  SampleTime=time_step
  "g_chosen " : Outport  Port=3  SampleTime=time_step
  f_chosen : Outport  Port=4  SampleTime=time_step
  largest hazard : Outport  Port=5  SampleTime=time_step
  smallest_hazard : Outport  Port=6  SampleTime=time_step
  "g_worst " : Outport  Port=7  SampleTime=time_step
  f_worst : Outport  Port=8  SampleTime=time_step
  psi_ca_worst : Outport  Port=9  SampleTime=time_step
  Pr_worst : Outport  Port=10  SampleTime=time_step
  scaled_mu_worst : Outport  Port=11  SampleTime=time_step
  R_worst : Outport  Port=12  SampleTime=time_step
  C_worst : Outport  Port=13  SampleTime=time_step
  chosen_scaled_mu : Outport  Port=14  SampleTime=time_step
  chosen_R : Outport  Port=15  SampleTime=time_step
  chosen_C : Outport  Port=16  SampleTime=time_step
  chosen_scenario_index : Outport  Port=17  SampleTime=time_step
  wires:
  SBMPC_obstacles_own_ship_x_predicted/1 -> Compute hazard/5(SBMPC_obstacles_own_ship_x_predicted)
  SBMPC_obstacles_own_ship_y_predicted/1 -> Compute hazard/6(SBMPC_obstacles_own_ship_y_predicted)
  obstacle_ships_x_predicted/1 -> Compute hazard/10(obstacle_ships_x_predicted_input)
  "obstacle_ships_y_predicted "/1 -> Compute hazard/11(obstacle_ships_y_predicted_input)
  t_0/1 -> Compute hazard/4(t_0)
  Compute hazard/1(CLOSE) -> To Workspace1/1
  Compute hazard/2(d_0) -> To Workspace2/1
  obstacle_ships_v/1 -> Compute hazard/2(obstacle_ships_v_input)
  obstacle_ships_u/1 -> Compute hazard/1(obstacle_ships_u_input)
  SBMPC_obstacles_own_ship_u_predicted/1 -> Compute hazard/7(SBMPC_obstacles_own_ship_u_predicted)
  "SBMPC_obstacles_own_ship_v_predicted "/1 -> Compute hazard/8(SBMPC_obstacles_own_ship_v_predicted)
  "SBMPC_obstacles_own_ship_heading_predicted "/1 -> Compute hazard/9(SBMPC_obstacles_own_ship_heading_predicted)
  obstacle_ships_psi/1 -> Compute hazard/3(obstacle_ships_psi_input)
  Compute hazard/3(OVERTAKEN) -> To Workspace3/1
  Compute hazard/4(STARBOARD) -> To Workspace4/1
  ? -> To Workspace5/1
  Compute hazard/6(CROSSED) -> To Workspace6/1
  Compute hazard/7(mu) -> To Workspace7/1
  Compute hazard/12(hazard) -> To Workspace12/1
  Compute hazard/8(C) -> To Workspace8/1
  Compute hazard/10(f) -> To Workspace10/1
  Compute hazard/11(g) -> To Workspace11/1
  Compute hazard/13(chosen_C_out) -> chosen_C/1, To Workspace13/1
  Compute hazard/16(chosen_R_out) -> To Workspace14/1, chosen_R/1
  Compute hazard/17(chosen_scaled_mu_out) -> To Workspace15/1, chosen_scaled_mu/1
  Compute hazard/19(chosen_psi_ca_out) -> To Workspace16/1, psi_ca/1
  Compute hazard/20(C_worst) -> To Workspace25/1, C_worst/1
  Compute hazard/21(R_worst) -> R_worst/1, To Workspace26/1
  Compute hazard/22(scaled_mu_worst) -> To Workspace27/1, scaled_mu_worst/1
  Compute hazard/23(Pr_worst) -> To Workspace29/1, Pr_worst/1
  Compute hazard/24(psi_ca_worst) -> psi_ca_worst/1, To Workspace28/1
  Compute hazard/26(g_worst_out) -> "g_worst "/1, To Workspace24/1
  Compute hazard/25(f_worst_out) -> f_worst/1, To Workspace23/1
  Compute hazard/18(chosen_Pr_out) -> To Workspace17/1, Pr/1
  Compute hazard/29(f_out) -> f_chosen/1, To Workspace18/1
  Compute hazard/30(g_out) -> "g_chosen "/1, To Workspace19/1
  Compute hazard/27(smallest_hazard_out) -> smallest_hazard/1, To Workspace20/1
  Compute hazard/28(largest_hazard_out) -> largest hazard/1, To Workspace21/1
  Compute hazard/9(R) -> Terminator/1
  Compute hazard/14(chosen_P_out) -> To Workspace9/1
  Compute hazard/15(chosen_FC_out) -> To Workspace30/1
  Compute hazard/31(chosen_scenario_index_out) -> To Workspace31/1, Scope/1, chosen_scenario_index/1

== system modules_intentions/SBMPC obstacle ships/SBMPC using intentions /Normal obstacle ships trajectories prediction ==
  note: column vector, row = time step in prediction horizion and column = obstacle
  note: column vector, row = time step in prediction horizion and column = obstacle
  t_0 : Inport
  normal_obstacle_ships_positions : Inport  Port=2
  normal_obstacle_ships_headings : Inport  Port=3
  normal_obstacle_ships_next_waypoints : Inport  Port=4
  Normal obstacle ships trajectories prediction : MATLAB Function  TreatAsAtomicUnit=on
  Scope1 : Scope
  To Workspace1 : ToWorkspace  Commented=on  VariableName=normal_obstacle_ships_u_predicted  SaveFormat=Structure With Time  SampleTime=tsamp
  To Workspace2 : ToWorkspace  Commented=on  VariableName=normal_obstacle_ships_psi_predicted  SaveFormat=Structure With Time  SampleTime=tsamp
  To Workspace3 : ToWorkspace  Commented=on  VariableName=normal_obstacle_ships_y_predicted  SaveFormat=Structure With Time  SampleTime=tsamp
  To Workspace4 : ToWorkspace  Commented=on  VariableName=normal_obstacle_ships_x_predicted  SaveFormat=Structure With Time  SampleTime=tsamp
  To Workspace5 : ToWorkspace  Commented=on  VariableName=normal_obstacle_ships_v_predicted  SaveFormat=Structure With Time  SampleTime=tsamp
  normal_obstacle_ships_x_predicted : Outport  SampleTime=time_step
  obstacle_ships_y_predicted : Outport  Port=2  SampleTime=time_step
  obstacle_ships_psi_predicted : Outport  Port=3  SampleTime=time_step
  obstacle_ships_u_predicted : Outport  Port=4  SampleTime=time_step
  obstacle_ships_v_predicted : Outport  Port=5  SampleTime=time_step
  wires:
  normal_obstacle_ships_positions/1 -> Normal obstacle ships trajectories prediction/3(obstacle_ships_initial_positions)
  t_0/1 -> Normal obstacle ships trajectories prediction/4(t_0)
  Normal obstacle ships trajectories prediction/1(obstacle_ships_x_predicted) -> normal_obstacle_ships_x_predicted/1, To Workspace4/1
  Normal obstacle ships trajectories prediction/2(obstacle_ships_y_predicted) -> obstacle_ships_y_predicted/1, To Workspace3/1
  normal_obstacle_ships_headings/1 -> Normal obstacle ships trajectories prediction/1(obstacle_ships_headings)
  normal_obstacle_ships_next_waypoints/1 -> Normal obstacle ships trajectories prediction/2(obstacle_ships_next_waypoint_index_vector), Scope1/1
  Normal obstacle ships trajectories prediction/5(obstacle_ships_psi_predicted) -> To Workspace2/1, obstacle_ships_psi_predicted/1
  Normal obstacle ships trajectories prediction/3(obstacle_ships_u_predicted) -> To Workspace1/1, obstacle_ships_u_predicted/1
  Normal obstacle ships trajectories prediction/4(obstacle_ships_v_predicted) -> To Workspace5/1, obstacle_ships_v_predicted/1
